simulink model "simproject"  (R2021b)
settings: Solver=VariableStepAuto  StartTime=0.0  StopTime=t_f  MaxStep=max_step  RelTol=1e-3
values from neighbouring files (symbols this model uses):
  Amplitude = 0.05    [Matlab_File.m]
  Anew = [    0                 1            0         0 ... (first row only)    [Matlab_File.m]
  B = [  0 ... (first row only)    [Matlab_File.m]
  C = [1 0 0 0]    [Matlab_File.m]
  D = 0    [Matlab_File.m]
  F = 0    [Matlab_File.m]
  K = X / W    [Matlab_File.m]
  phi_cosine = pi/3    (= 1.0471975512)    [Matlab_File.m]
  phi_sine = 0    [Matlab_File.m]
  w_cosine = 30    [Matlab_File.m]
  w_sine = 80    [Matlab_File.m]
  x0 = [0; 0; 0; 0]    [Matlab_File.m]
settings Model: Creator=loren  LastModifiedBy=loren
settings DataIOCC: ReturnWorkspaceOutputs=off

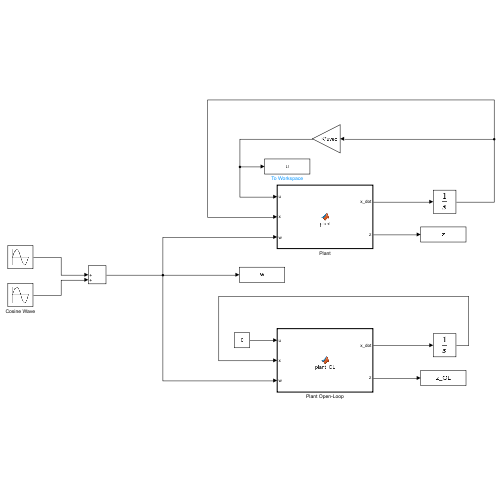
[thumbnail: Simulink's stored preview of the top-level diagram]
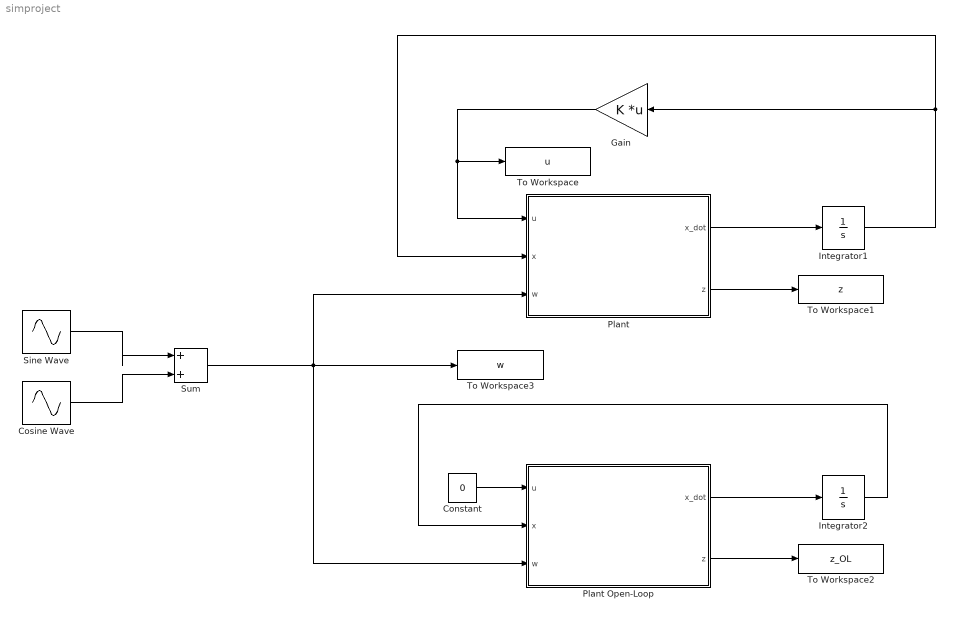
== system simproject ==
  Constant : Constant  Value=0
  Cosine Wave : Sin  Amplitude=Amplitude  Frequency=w_cosine  Phase=phi_cosine+(pi/2)  SampleTime=0
  Gain : Gain  Gain=K  Multiplication=Matrix(K*u) (u vector)
  Integrator1 : Integrator  InitialCondition=x0
  Integrator2 : Integrator  InitialCondition=x0
  Plant : MATLAB Function  TreatAsAtomicUnit=on
  Plant Open-Loop : MATLAB Function  TreatAsAtomicUnit=on
  Sine Wave : Sin  Amplitude=Amplitude  Frequency=w_sine  Phase=phi_sine  SampleTime=0
  Sum : Sum  Inputs=|++
  To Workspace : ToWorkspace  VariableName=u  SaveFormat=Timeseries  SampleTime=-1
  To Workspace1 : ToWorkspace  VariableName=z  SampleTime=-1
  To Workspace2 : ToWorkspace  VariableName=z_OL  SampleTime=-1
  To Workspace3 : ToWorkspace  VariableName=w  SaveFormat=Timeseries  SampleTime=-1
  wires:
  Gain/1 -> To Workspace/1, Plant/1(u)
  Integrator2/1 -> Plant Open-Loop/2(x)
  Constant/1 -> Plant Open-Loop/1(u)
  Plant/1(x_dot) -> Integrator1/1
  Integrator1/1 -> Gain/1, Plant/2(x)
  Plant Open-Loop/2(z) -> To Workspace2/1
  Plant Open-Loop/1(x_dot) -> Integrator2/1
  Plant/2(z) -> To Workspace1/1
  Sine Wave/1 -> Sum/1
  Cosine Wave/1 -> Sum/2
  Sum/1 -> Plant/3(w), To Workspace3/1, Plant Open-Loop/3(w)

== matlab function simproject/Plant ==
  data: u input; x_dot output; x input; w input; z output; Anew parameter; B parameter; C parameter; D parameter; E parameter; F parameter
function [x_dot, z] = plant(u, x, w, Anew, B, C, D, E, F)

x_dot = Anew*x + B*u + E*w;
z = C*x + D*u + F*w;

== matlab function simproject/Plant Open-Loop ==
  data: u input; x_dot output; x input; w input; z output; Anew parameter; B parameter; C parameter; D parameter; E parameter; F parameter
function [x_dot, z] = plant_OL(u, x, w, Anew, B, C, D, E, F)

x_dot = Anew*x + B*u + E*w;
z = C*x + D*u + F*w;
